simulink model "trap_mf"  (Simulink 7.2)
settings: Solver=ode45  StartTime=0.0  StopTime=10.0  RelTol=1e-3
values from neighbouring files (symbols this model uses):
  fi_1_a = -0.786    [fuzzy_controller_3_trimf_params.m]    (also in fuzzy_controller_5_gbell_params.m = 0.1768; fuzzy_controller_5_trimf_optimal_params.m; fuzzy_controller_5_trimf_params.m; fuzzy_controller_7_trimf_params.m)
  fi_1_b = -0.786    [fuzzy_controller_3_trimf_params.m]    (also in fuzzy_controller_5_gbell_params.m = 3.278; fuzzy_controller_5_trimf_optimal_params.m; fuzzy_controller_5_trimf_params.m; fuzzy_controller_7_trimf_params.m)
  fi_1_c = 0    [fuzzy_controller_3_trimf_params.m]    (also in fuzzy_controller_5_gbell_params.m = -0.7664; fuzzy_controller_5_trimf_optimal_params.m = -0.1; fuzzy_controller_5_trimf_params.m = -0.393; fuzzy_controller_7_trimf_params.m = -0.523)
  fi_1_d = -0.05    [fuzzy_controller_5_trimf_optimal_params.m]
settings Model: Creator=Student  ModifiedByFormat=Student  LastModifiedBy=Student
settings OptimizationCC: ExpressionDepthLimit=128
settings DebuggingCC: AlgebraicLoopMsg=error  UnderspecifiedInitializationDetection=Simplified  MergeDetectMultiDrivingBlocksExec=error  SolverPrmCheckMsg=none  FcnCallInpInsideContextMsg=Enable All  StateNameClashWarn=none  StrictBusMsg=ErrorLevel1
settings HardwareCC: ProdBitPerLong=64  ProdIntDivRoundTo=Zero  ProdEndianess=LittleEndian  ProdWordSize=64  ProdHWDeviceType=Intel->x86-64
settings RTWCC: Description=Create Visual C/C++ Solution File for Simulink Coder  GenerateReport=on  RetainRTWFile=on  LaunchReport=on
settings CodeAppCC: ForceParamTrailComments=on  CustomSymbolStrType=$N$R$M_T
settings GRTTargetCC: TargetFunctionLibrary=C99 (ISO)

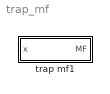
== system trap_mf ==
  trap mf1 : Subsystem  mask{a=fi_1_a, b=fi_1_b, c=fi_1_c, d=fi_1_d}
      mask prompts: a "Left base point a:"; b "Left peak location b:"; c "Right base point c:"; d "Right peak location d:"

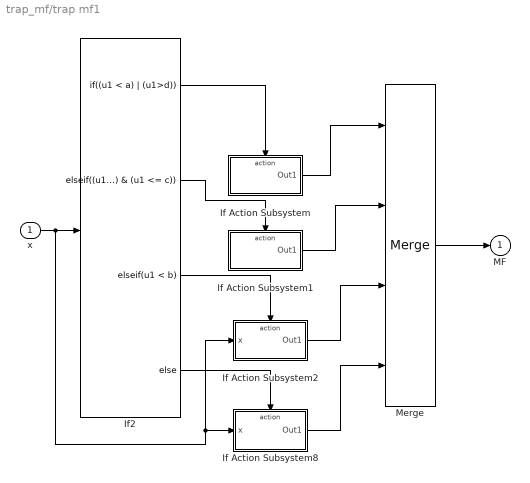
== system trap_mf/trap mf1 ==
  x : Inport
  If Action Subsystem : Subsystem  TreatAsAtomicUnit=on
  If Action Subsystem1 : Subsystem  TreatAsAtomicUnit=on
  If Action Subsystem2 : Subsystem  TreatAsAtomicUnit=on
  If Action Subsystem8 : Subsystem  TreatAsAtomicUnit=on
  If2 : If  IfExpression=(u1 < a) | (u1>d)  ElseIfExpressions=(u1 >= b) & (u1 <= c), u1 < b  ZeroCross=off
  Merge : Merge  Inputs=4  InitialOutput=0
  MF : Outport
  wires:
  If Action Subsystem2/1(Out1) -> Merge/3
  If2/3 -> If Action Subsystem2/Action
  If Action Subsystem8/1(Out1) -> Merge/4
  If2/4 -> If Action Subsystem8/Action
  If Action Subsystem1/1(Out1) -> Merge/2
  If2/2 -> If Action Subsystem1/Action
  If Action Subsystem/1(Out1) -> Merge/1
  Merge/1 -> MF/1
  If2/1 -> If Action Subsystem/Action
  x/1 -> If Action Subsystem2/1(x), If Action Subsystem8/1(x), If2/1

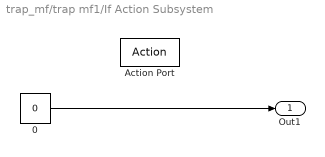
== system trap_mf/trap mf1/If Action Subsystem ==
  Action Port : ActionPort
  0 : Constant  Value=0
  Out1 : Outport  InitialOutput=0
  wires:
  0/1 -> Out1/1

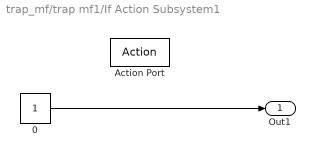
== system trap_mf/trap mf1/If Action Subsystem1 ==
  Action Port : ActionPort
  0 : Constant
  Out1 : Outport  InitialOutput=1
  wires:
  0/1 -> Out1/1

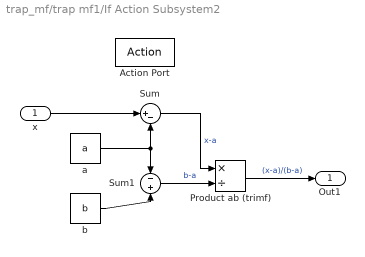
== system trap_mf/trap mf1/If Action Subsystem2 ==
  x : Inport
  Action Port : ActionPort
  Product ab (trimf) : Product  Inputs=*/  SampleTime=[0 1]  SaturateOnIntegerOverflow=on  InputSameDT=on  OutDataTypeStr=Inherit: Same as first input
  Sum : Sum  Inputs=|+-  SaturateOnIntegerOverflow=on  InputSameDT=on  OutDataTypeStr=Inherit: Same as first input
  Sum1 : Sum  Inputs=-+  SaturateOnIntegerOverflow=on  InputSameDT=on  OutDataTypeStr=Inherit: Same as first input
  a : Constant  Value=a
  b : Constant  Value=b
  Out1 : Outport
  wires:
  Sum1/1 -> Product ab (trimf)/2  "b-a"
  Sum/1 -> Product ab (trimf)/1  "x-a"
  x/1 -> Sum/1
  b/1 -> Sum1/2
  a/1 -> Sum1/1, Sum/2
  Product ab (trimf)/1 -> Out1/1  "(x-a)/(b-a)"

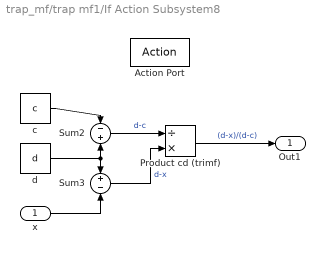
== system trap_mf/trap mf1/If Action Subsystem8 ==
  x : Inport
  Action Port : ActionPort
  Product cd (trimf) : Product  Inputs=/*  SampleTime=[0 1]  SaturateOnIntegerOverflow=on  InputSameDT=on  OutDataTypeStr=Inherit: Same as first input
  Sum2 : Sum  Inputs=-+  SaturateOnIntegerOverflow=on  InputSameDT=on  OutDataTypeStr=Inherit: Same as first input
  Sum3 : Sum  Inputs=+-  SaturateOnIntegerOverflow=on  InputSameDT=on  OutDataTypeStr=Inherit: Same as first input
  c : Constant  Value=c
  d : Constant  Value=d
  Out1 : Outport
  wires:
  c/1 -> Sum2/1
  x/1 -> Sum3/2
  d/1 -> Sum3/1, Sum2/2
  Sum3/1 -> Product cd (trimf)/2  "d-x"
  Sum2/1 -> Product cd (trimf)/1  "d-c"
  Product cd (trimf)/1 -> Out1/1  "(d-x)/(d-c)"
